simulink model "sampleModel1513"  (R2023a)
settings: Solver=VariableStepAuto  StartTime=0.0  StopTime=10.0  RelTol=1e-3
libraries: hdlsllib x2, simulink x1
settings Model: Creator=user1  LastModifiedBy=user1

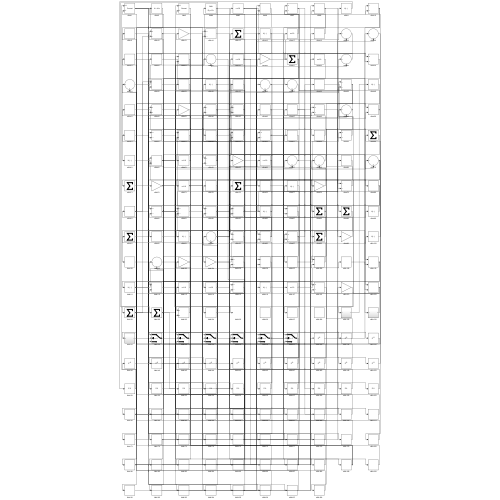
[thumbnail: Simulink's stored preview of the top-level diagram]
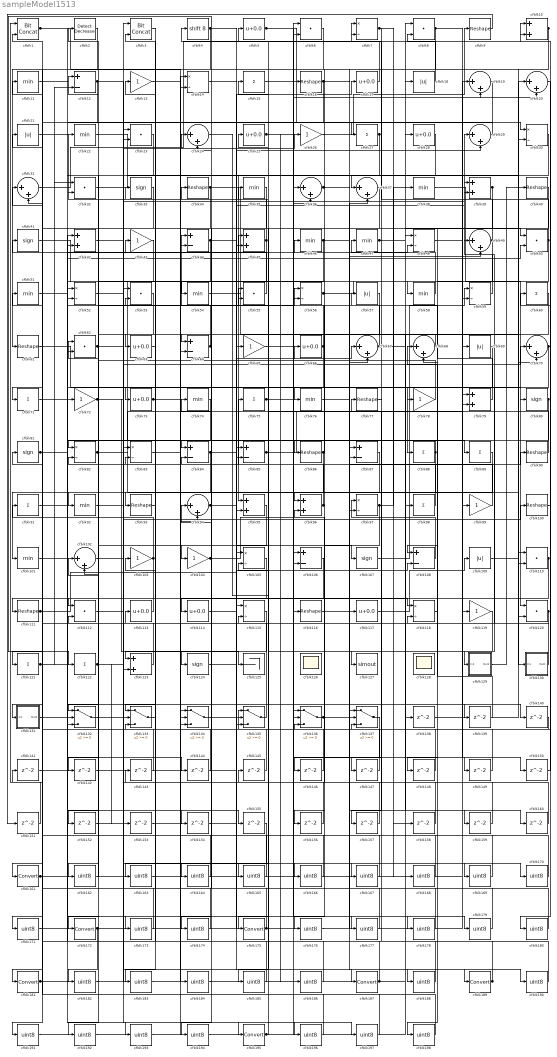
== system sampleModel1513 ==
  cfblk1 : hdlsllib/Logic and Bit Operations/Bit Concat  numInputs=2
  cfblk{10,39,42,45,79,95..96,123} (8 alike) : Sum
  cfblk{9,16,34,40,61,77,86,90,93,100,111,116} (12 alike) : Reshape
  cfblk{11,22,35,38,46..47,51,54,58,74,76,92,101} (13 alike) : MinMax
  cfblk{19..20,24,29,31,36..37,49,67..68,70,94,102} (13 alike) : Sum  Inputs=|++
  cfblk{13,26,43,65,72,78,99,103..104,119} (10 alike) : Gain
  cfblk{7,14,30,48,52,56,59,82..83,97,105,115,118} (13 alike) : Product  Inputs=*/  RndMeth=Zero  SaturateOnIntegerOverflow=on
  cfblk{12,44,64,84..85,87,106,108} (8 alike) : Sum  Inputs=+-
  cfblk{33,41,80..81,107,124} (6 alike) : Signum
  cfblk{18,21,57,69,109} (5 alike) : Abs  SaturateOnIntegerOverflow=off
  cfblk{6,8,23,32,50,53,55,62,110,112,120} (11 alike) : DotProduct  OutDataTypeStr=Inherit: Inherit via internal rule
  cfblk{5,17,25,28,63,66,73,113..114,117} (10 alike) : Bias  Bias=0.0  SaturateOnIntegerOverflow=off
  cfblk{15,27,60,71,75,88..89,91,98,121..122} (11 alike) : Sum  Inputs=+
  cfblk125 : Terminator
  cfblk126 : Scope
      settings: Floating=on
  cfblk127 : ToWorkspace  VariableName=simout  SaveFormat=Timeseries  SampleTime=-1
  cfblk128 : Scope
      settings: Floating=on
  cfblk129 : Subsystem
      settings: LibrarySourceBlock=|
      | hdlsllib/Ports &
      | Subsystems/Subsystem
  cfblk130 : Subsystem
      settings: LibrarySourceBlock=|
      | hdlsllib/Ports &
      | Subsystems/Subsystem
  cfblk131 : Subsystem
      settings: LibrarySourceBlock=|
      | hdlsllib/Ports &
      | Subsystems/Subsystem
  cfblk{132..137} (6 alike) : Switch  SaturateOnIntegerOverflow=off  InputSameDT=off
  cfblk{138..160} (23 alike) : Delay  SampleTime=1
  cfblk{161,172,175,181,187,189,195} (7 alike) : DataTypeConversion  SaturateOnIntegerOverflow=off  RndMeth=Floor
  cfblk{162..171,173..174,176..180,182..186,188,190..194,196..198} (31 alike) : DataTypeConversion  OutDataTypeStr=uint8  SaturateOnIntegerOverflow=off  RndMeth=Floor
  cfblk2 : simulink/Logic and Bit Operations/Detect Decrease  vinit=0.0  OutDataTypeStr=boolean
      settings: LibrarySourceBlock=|
      | hdlsllib/Logic and Bit
      | Operations/Detect
      | Decrease
  cfblk3 : hdlsllib/Logic and Bit Operations/Bit Concat  numInputs=2
  cfblk4 : ArithShift  BitShiftNumber=8
  wires:
  cfblk107/1 -> cfblk59/1
  cfblk58/1 -> cfblk47/1
  cfblk129/1(Out1) -> cfblk40/1
  cfblk13/1 -> cfblk187/1
  cfblk27/1 -> cfblk95/1, cfblk162/1
  cfblk4/1 -> cfblk61/1, cfblk107/1
  cfblk60/1 -> cfblk95/2
  cfblk24/1 -> cfblk113/1
  cfblk72/1 -> cfblk125/1, cfblk70/1
  cfblk94/1 -> cfblk66/1, cfblk56/2, cfblk39/2
  cfblk17/1 -> cfblk122/1
  cfblk53/1 -> cfblk172/1
  cfblk43/1 -> cfblk84/1
  cfblk26/1 -> cfblk9/1
  cfblk45/1 -> cfblk22/1, cfblk124/1
  cfblk2/1 -> cfblk161/1
  cfblk6/1 -> cfblk181/1
  cfblk88/1 -> cfblk127/1, cfblk86/1
  cfblk84/1 -> cfblk93/1, cfblk29/2, cfblk170/1
  cfblk87/1 -> cfblk101/1
  cfblk14/1 -> cfblk189/1
  cfblk18/1 -> cfblk8/2
  cfblk56/1 -> cfblk58/1, cfblk67/2
  cfblk59/1 -> cfblk29/1
  cfblk133/1 -> cfblk103/1
  cfblk23/1 -> cfblk82/1
  cfblk115/1 -> cfblk123/1
  cfblk38/1 -> cfblk120/1
  cfblk35/1 -> cfblk114/1
  cfblk111/1 -> cfblk65/1, cfblk55/2
  cfblk93/1 -> cfblk133/1
  cfblk98/1 -> cfblk62/1
  cfblk92/1 -> cfblk26/1
  cfblk119/1 -> cfblk175/1
  cfblk8/1 -> cfblk30/1, cfblk87/2
  cfblk41/1 -> cfblk79/1
  cfblk135/1 -> cfblk74/1
  cfblk67/1 -> cfblk32/2, cfblk159/1
  cfblk65/1 -> cfblk136/1
  cfblk71/1 -> cfblk72/1
  cfblk80/1 -> cfblk85/2, cfblk164/1
  cfblk25/1 -> cfblk149/1, cfblk186/1
  cfblk5/1 -> cfblk99/1, cfblk79/2, cfblk70/2
  cfblk49/1 -> cfblk7/1, cfblk108/1
  cfblk109/1 -> cfblk130/1(In1)
  cfblk69/1 -> cfblk76/1
  cfblk78/1 -> cfblk12/1
  cfblk62/1 -> cfblk24/1, cfblk139/1, cfblk188/1
  cfblk97/1 -> cfblk38/1, cfblk156/1
  cfblk61/1 -> cfblk88/1
  cfblk12/1 -> cfblk71/1, cfblk154/1
  cfblk47/1 -> cfblk50/1, cfblk168/1
  cfblk7/1 -> cfblk157/1, cfblk158/1
  cfblk31/1 -> cfblk10/1
  cfblk103/1 -> cfblk31/2, cfblk121/1
  cfblk36/1 -> cfblk78/1, cfblk176/1
  cfblk113/1 -> cfblk112/1
  cfblk19/1 -> cfblk52/2
  cfblk64/1 -> cfblk44/1, cfblk44/2
  cfblk79/1 -> cfblk57/1
  cfblk34/1 -> cfblk116/1, cfblk171/1
  cfblk20/1 -> cfblk135/1
  cfblk96/1 -> cfblk75/1, cfblk24/2
  cfblk74/1 -> cfblk132/1
  cfblk32/1 -> cfblk37/1
  cfblk29/1 -> cfblk27/1
  cfblk124/1 -> cfblk67/1
  cfblk91/1 -> cfblk195/1
  cfblk63/1 -> cfblk33/1
  cfblk30/1 -> cfblk62/2
  cfblk54/1 -> cfblk98/1
  cfblk66/1 -> cfblk43/1, cfblk132/3, cfblk194/1
  cfblk81/1 -> cfblk32/1, cfblk155/1
  cfblk104/1 -> cfblk16/1, cfblk108/2
  cfblk46/1 -> cfblk64/1, cfblk190/1
  cfblk123/1 -> cfblk41/1
  cfblk120/1 -> cfblk112/2, cfblk118/2
  cfblk10/1 -> cfblk96/1, cfblk110/2
  cfblk44/1 -> cfblk92/1, cfblk17/1
  cfblk108/1 -> cfblk97/1
  cfblk86/1 -> cfblk56/1, cfblk104/1
  cfblk55/1 -> cfblk21/1
  cfblk130/1(Out1) -> cfblk49/1
  cfblk90/1 -> cfblk55/1
  cfblk122/1 -> cfblk100/1, cfblk153/1
  cfblk40/1 -> cfblk73/1
  cfblk22/1 -> cfblk110/1
  cfblk75/1 -> cfblk20/2, cfblk80/1
  cfblk117/1 -> cfblk109/1
  cfblk1/1 -> cfblk94/2, cfblk30/2, cfblk54/1, cfblk89/1
  cfblk33/1 -> cfblk111/1
  cfblk82/1 -> cfblk19/1, cfblk120/2, cfblk178/1
  cfblk110/1 -> cfblk131/1(In1), cfblk134/3
  cfblk39/1 -> cfblk68/2, cfblk59/2
  cfblk76/1 -> cfblk137/1
  cfblk70/1 -> cfblk129/1(In1), cfblk180/1, cfblk185/1
  cfblk99/1 -> cfblk35/1
  cfblk136/1 -> cfblk90/1, cfblk49/2
  cfblk28/1 -> cfblk137/2
  cfblk132/1 -> cfblk39/1
  cfblk85/1 -> cfblk36/2, cfblk19/2
  cfblk100/1 -> cfblk60/1
  cfblk114/1 -> cfblk48/2
  cfblk68/1 -> cfblk63/1
  cfblk21/1 -> cfblk134/2
  cfblk121/1 -> cfblk45/1, cfblk12/2, cfblk50/2
  cfblk50/1 -> cfblk7/2, cfblk198/1
  cfblk116/1 -> cfblk37/2
  cfblk16/1 -> cfblk45/2, cfblk160/1
  cfblk73/1 -> cfblk118/1, cfblk46/1
  cfblk138/1 -> cfblk20/1
  cfblk139/1 -> cfblk68/1
  cfblk112/1 -> cfblk140/1
  cfblk140/1 -> cfblk136/3
  cfblk141/1 -> cfblk115/1
  cfblk105/1 -> cfblk142/1
  cfblk142/1 -> cfblk134/1
  cfblk143/1 -> cfblk1/2
  cfblk101/1 -> cfblk144/1
  cfblk144/1 -> cfblk31/1
  cfblk145/1 -> cfblk132/2
  cfblk137/1 -> cfblk146/1
  cfblk146/1 -> cfblk94/1
  cfblk77/1 -> cfblk147/1
  cfblk147/1 -> cfblk23/1
  cfblk118/1 -> cfblk148/1
  cfblk148/1 -> cfblk133/3
  cfblk149/1 -> cfblk82/2
  cfblk48/1 -> cfblk150/1
  cfblk150/1 -> cfblk10/2
  cfblk9/1 -> cfblk151/1
  cfblk151/1 -> cfblk1/1
  cfblk95/1 -> cfblk152/1
  cfblk152/1 -> cfblk123/2
  cfblk153/1 -> cfblk135/3
  cfblk154/1 -> cfblk135/2
  cfblk156/1 -> cfblk133/2
  cfblk157/1 -> cfblk136/2
  cfblk158/1 -> cfblk96/2
  cfblk159/1 -> cfblk84/2
  cfblk160/1 -> cfblk4/1
  cfblk161/1 -> cfblk64/2, cfblk69/1, cfblk117/1
  cfblk162/1 -> cfblk2/1
  cfblk3/1 -> cfblk163/1
  cfblk163/1 -> cfblk36/1
  cfblk164/1 -> cfblk3/1
  cfblk37/1 -> cfblk165/1
  cfblk165/1 -> cfblk3/2
  cfblk102/1 -> cfblk166/1
  cfblk166/1 -> cfblk115/2
  cfblk134/1 -> cfblk167/1
  cfblk167/1 -> cfblk102/1
  cfblk168/1 -> cfblk102/2
  cfblk42/1 -> cfblk169/1
  cfblk169/1 -> cfblk81/1
  cfblk170/1 -> cfblk42/1
  cfblk171/1 -> cfblk42/2
  cfblk172/1 -> cfblk85/1, cfblk97/2, cfblk182/1
  cfblk131/1(Out1) -> cfblk173/1
  cfblk173/1 -> cfblk53/1
  cfblk57/1 -> cfblk174/1
  cfblk174/1 -> cfblk53/2
  cfblk175/1 -> cfblk87/1, cfblk105/1, cfblk28/1
  cfblk176/1 -> cfblk119/1
  cfblk15/1 -> cfblk177/1
  cfblk177/1 -> cfblk34/1
  cfblk178/1 -> cfblk15/1
  cfblk11/1 -> cfblk179/1
  cfblk179/1 -> cfblk77/1
  cfblk180/1 -> cfblk11/1
  cfblk181/1 -> cfblk138/1, cfblk23/2, cfblk193/1
  cfblk182/1 -> cfblk6/1
  cfblk155/1 -> cfblk183/1
  cfblk183/1 -> cfblk6/2
  cfblk83/1 -> cfblk184/1
  cfblk184/1 -> cfblk48/1
  cfblk185/1 -> cfblk83/1
  cfblk186/1 -> cfblk83/2
  cfblk187/1 -> cfblk143/1, cfblk141/1, cfblk105/2
  cfblk188/1 -> cfblk13/1
  cfblk189/1 -> cfblk137/3, cfblk25/1, cfblk52/1
  cfblk190/1 -> cfblk14/1
  cfblk89/1 -> cfblk191/1
  cfblk191/1 -> cfblk14/2
  cfblk106/1 -> cfblk192/1
  cfblk192/1 -> cfblk8/1
  cfblk193/1 -> cfblk106/1
  cfblk194/1 -> cfblk106/2
  cfblk195/1 -> cfblk145/1, cfblk18/1
  cfblk52/1 -> cfblk196/1
  cfblk196/1 -> cfblk91/1
  cfblk51/1 -> cfblk197/1
  cfblk197/1 -> cfblk5/1
  cfblk198/1 -> cfblk51/1

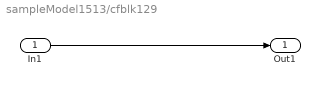
== system sampleModel1513/cfblk129 ==
  In1 : Inport
  Out1 : Outport
  wires:
  In1/1 -> Out1/1

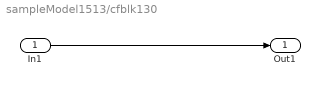
== system sampleModel1513/cfblk130 ==
  In1 : Inport
  Out1 : Outport
  wires:
  In1/1 -> Out1/1

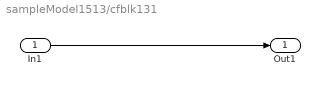
== system sampleModel1513/cfblk131 ==
  In1 : Inport
  Out1 : Outport
  wires:
  In1/1 -> Out1/1
